simulink model "DReqSwt_DD"  (R2016b)
settings: configuration reference "CodeGenConfigSet" (kept outside this file)
values from neighbouring files (symbols this model uses):
  DReqSwt_tiDebClrHiLo_C = Calibration.Parameter    [init_DReqSwt_DD.m]
  DReqSwt_tiDebClrLoHi_C = Calibration.Parameter    [init_DReqSwt_DD.m]
  DReqSwt_tiDebHiLo_C = Calibration.Parameter    [init_DReqSwt_DD.m]
  DReqSwt_tiDebLoHi_C = Calibration.Parameter    [init_DReqSwt_DD.m]
undefined symbols (not defined in the file or in its folder): DReqSwt_DD_DT
libraries: CXLib x2
settings Model: Creator=xinchangran  LastModifiedBy=xinchangran
settings ConfigSetRef: SourceLocation=Base Workspace

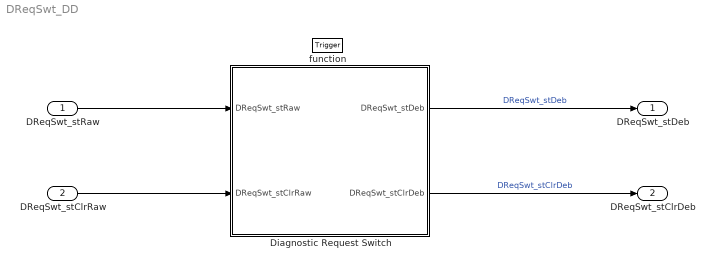
== system DReqSwt_DD ==
  DReqSwt_stRaw : Inport  Description=Diagnostic Request Switch  OutMin=0  OutMax=1  OutDataTypeStr=boolean
  DReqSwt_stClrRaw : Inport  Description=Diagnostic Memory Clear Switch  Port=2  OutMin=0  OutMax=1  OutDataTypeStr=boolean
  function : TriggerPort  TriggerType=function-call  VariantControl=Variant
  Diagnostic Request Switch : Subsystem
  DReqSwt_stDeb : Outport  Description="after debounced status  Switch"  OutMin=0  OutMax=1  OutDataTypeStr=boolean
  DReqSwt_stClrDeb : Outport  Description=after debounced status Clear Switch  Port=2  OutMin=0  OutMax=1  OutDataTypeStr=boolean
  wires:
  DReqSwt_stRaw/1 -> Diagnostic Request Switch/1(DReqSwt_stRaw)
  DReqSwt_stClrRaw/1 -> Diagnostic Request Switch/2(DReqSwt_stClrRaw)
  Diagnostic Request Switch/1(DReqSwt_stDeb) -> DReqSwt_stDeb/1  "DReqSwt_stDeb"
  Diagnostic Request Switch/2(DReqSwt_stClrDeb) -> DReqSwt_stClrDeb/1  "DReqSwt_stClrDeb"

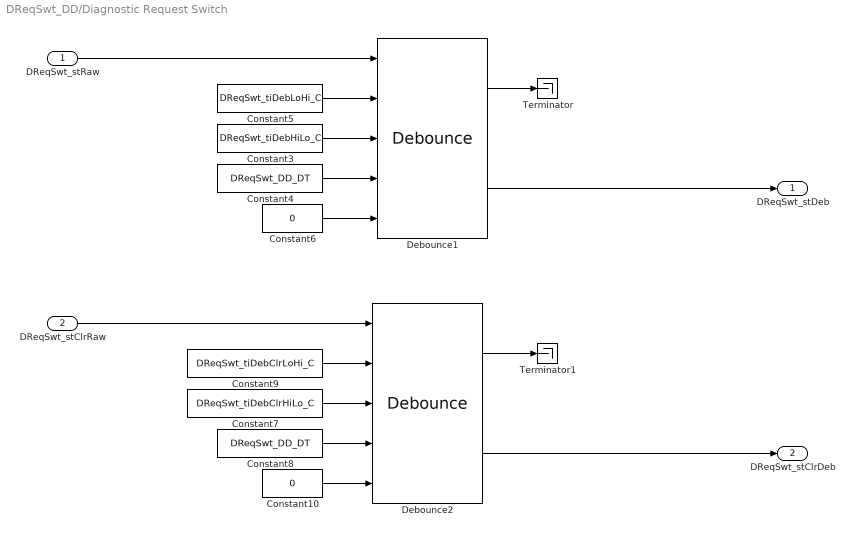
== system DReqSwt_DD/Diagnostic Request Switch ==
  DReqSwt_stRaw : Inport  Description=Diagnostic Request Switch  OutMin=0  OutMax=1  OutDataTypeStr=boolean
  DReqSwt_stClrRaw : Inport  Description=Diagnostic Memory Clear Switch  Port=2  OutMin=0  OutMax=1  OutDataTypeStr=boolean
  Constant10 : Constant  Value=0  OutDataTypeStr=Inherit: Inherit via back propagation
  Constant3 : Constant  Value=DReqSwt_tiDebHiLo_C
  Constant4 : Constant  Value=DReqSwt_DD_DT
  Constant5 : Constant  Value=DReqSwt_tiDebLoHi_C
  Constant6 : Constant  Value=0  OutDataTypeStr=Inherit: Inherit via back propagation
  Constant7 : Constant  Value=DReqSwt_tiDebClrHiLo_C
  Constant8 : Constant  Value=DReqSwt_DD_DT
  Constant9 : Constant  Value=DReqSwt_tiDebClrLoHi_C
  Debounce1 : CXLib/Debounce
  Debounce2 : CXLib/Debounce
  Terminator : Terminator
  Terminator1 : Terminator
  DReqSwt_stDeb : Outport  Description="after debounced status  Switch"  OutMin=0  OutMax=1  OutDataTypeStr=boolean
  DReqSwt_stClrDeb : Outport  Description=after debounced status Clear Switch  Port=2  OutMin=0  OutMax=1  OutDataTypeStr=boolean
  wires:
  Constant3/1 -> Debounce1/3
  Constant6/1 -> Debounce1/5
  Constant7/1 -> Debounce2/3
  Constant5/1 -> Debounce1/2
  Constant8/1 -> Debounce2/4
  DReqSwt_stRaw/1 -> Debounce1/1
  Constant4/1 -> Debounce1/4
  Constant9/1 -> Debounce2/2
  Constant10/1 -> Debounce2/5
  DReqSwt_stClrRaw/1 -> Debounce2/1
  Debounce1/1 -> Terminator/1
  Debounce2/1 -> Terminator1/1
  Debounce1/2 -> DReqSwt_stDeb/1
  Debounce2/2 -> DReqSwt_stClrDeb/1
